simulink model "PID_Tun"  (R2018a)
settings: Solver=ode5  StartTime=0.0  StopTime=T_stop  FixedStep=Ts  RelTol=1e-3
values from neighbouring files (symbols this model uses):
  Kd = str2num(get(handles.editPID_Kd,'string'))    [SCARA1.m]    (also in SavePID.mat = 0; TunPID.mat = 1)
  Ki = str2num(get(handles.editPID_Ki,'string'))    [SCARA1.m]    (also in SavePID.mat = 0; TunPID.mat = 0.1)
  Kp = str2num(get(handles.editPID_Kp,'string'))    [SCARA1.m]    (also in SavePID.mat = 1; TunPID.mat = 5)
settings Model: Creator=ASUS  LastModifiedBy=ASUS
settings DataIOCC: SaveFormat=Structure  ReturnWorkspaceOutputs=on  OutputSaveName=theta

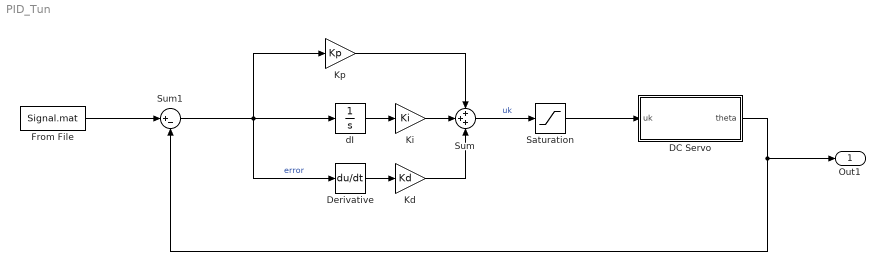
== system PID_Tun ==
  DC Servo : Subsystem  mask{K=1, Tu=0.1, Tm=0.2}
  Derivative : Derivative
  From File : FromFile  FileName=Signal.mat  SampleTime=0
  Kd : Gain  Gain=Kd
  Ki : Gain  Gain=Ki
  Kp : Gain  Gain=Kp
  Saturation : Saturate  UpperLimit=12  LowerLimit=-12
  Sum : Sum  Inputs=3
  Sum1 : Sum  Inputs=|+-
  dI : Integrator
  Out1 : Outport
  wires:
  Sum/1 -> Saturation/1  "uk"
  Ki/1 -> Sum/2
  Kd/1 -> Sum/3
  Kp/1 -> Sum/1
  DC Servo/1(theta) -> Out1/1, Sum1/2
  From File/1 -> Sum1/1
  Sum1/1 -> Kp/1, Derivative/1, dI/1  "error"
  Saturation/1 -> DC Servo/1(uk)
  dI/1 -> Ki/1
  Derivative/1 -> Kd/1

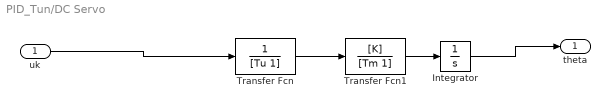
== system PID_Tun/DC Servo ==
  uk : Inport
  Integrator : Integrator
  Transfer Fcn : TransferFcn  Denominator=[Tu 1]
  Transfer Fcn1 : TransferFcn  Numerator=[K]  Denominator=[Tm 1]
  theta : Outport
  wires:
  Transfer Fcn/1 -> Transfer Fcn1/1
  Integrator/1 -> theta/1
  Transfer Fcn1/1 -> Integrator/1
  uk/1 -> Transfer Fcn/1
